simulink model "zadacha_14"  (Simulink 7.1)
settings: Solver=ode45  StartTime=0.0  StopTime=160  RelTol=1e-3
settings Model: Creator=Slavi  LastModifiedBy=Slavi

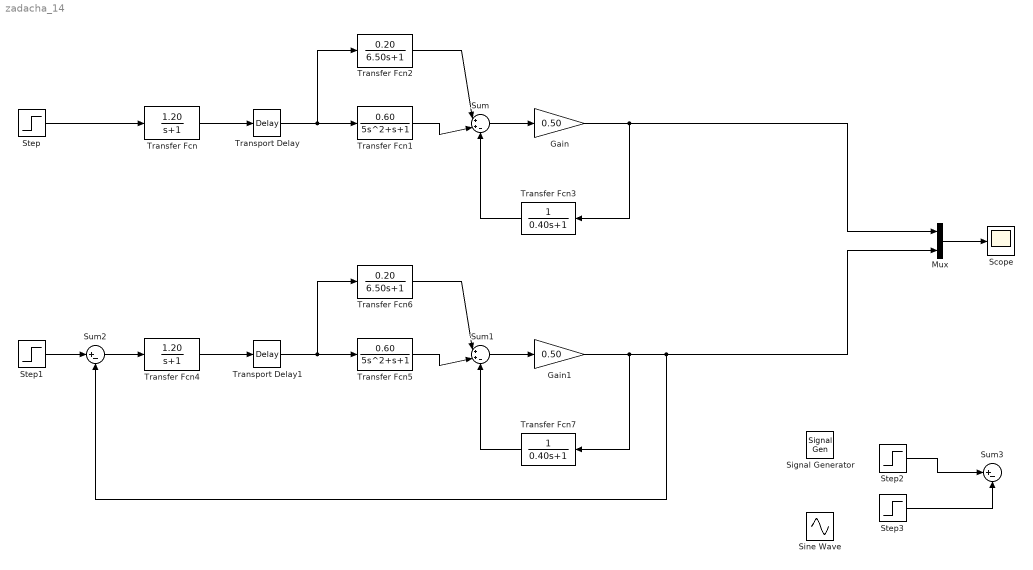
== system zadacha_14 ==
  Gain : Gain  Gain=0.50  ParameterDataType=sfix(16)  ParameterScaling=2^0  OutDataType=sfix(16)  OutScaling=2^0
  Gain1 : Gain  Gain=0.50  ParameterDataType=sfix(16)  ParameterScaling=2^0  OutDataType=sfix(16)  OutScaling=2^0
  Mux : Mux  Inputs=2
  Scope : Scope
  Signal Generator : SignalGenerator
  Sine Wave : Sin
  Step : Step
  Step1 : Step
  Step2 : Step  Time=0
  Step3 : Step
  Sum : Sum  Inputs=|++-  OutDataType=sfix(16)  OutScaling=2^0
  Sum1 : Sum  Inputs=|++-  OutDataType=sfix(16)  OutScaling=2^0
  Sum2 : Sum  Inputs=|+-  OutDataType=sfix(16)  OutScaling=2^0
  Sum3 : Sum  Inputs=|+-  OutDataType=sfix(16)  OutScaling=2^0
  Transfer Fcn : TransferFcn  Numerator=[1.20]  Denominator=[1 1]
  Transfer Fcn1 : TransferFcn  Numerator=[0.60]  Denominator=[5 1 1]
  Transfer Fcn2 : TransferFcn  Numerator=[0.20]  Denominator=[6.50 1]
  Transfer Fcn3 : TransferFcn  Orientation=left  Denominator=[0.40 1]
  Transfer Fcn4 : TransferFcn  Numerator=[1.20]  Denominator=[1 1]
  Transfer Fcn5 : TransferFcn  Numerator=[0.60]  Denominator=[5 1 1]
  Transfer Fcn6 : TransferFcn  Numerator=[0.20]  Denominator=[6.50 1]
  Transfer Fcn7 : TransferFcn  Orientation=left  Denominator=[0.40 1]
  Transport Delay : TransportDelay  DelayTime=2.40
  Transport Delay1 : TransportDelay  DelayTime=2.40
  wires:
  Transfer Fcn/1 -> Transport Delay/1
  Transport Delay/1 -> Transfer Fcn1/1, Transfer Fcn2/1
  Transfer Fcn1/1 -> Sum/2
  Transfer Fcn2/1 -> Sum/1
  Transfer Fcn3/1 -> Sum/3
  Sum/1 -> Gain/1
  Gain/1 -> Transfer Fcn3/1, Mux/1
  Mux/1 -> Scope/1
  Transfer Fcn4/1 -> Transport Delay1/1
  Transport Delay1/1 -> Transfer Fcn5/1, Transfer Fcn6/1
  Transfer Fcn5/1 -> Sum1/2
  Transfer Fcn6/1 -> Sum1/1
  Transfer Fcn7/1 -> Sum1/3
  Sum1/1 -> Gain1/1
  Gain1/1 -> Transfer Fcn7/1, Mux/2, Sum2/2
  Sum2/1 -> Transfer Fcn4/1
  Step2/1 -> Sum3/1
  Step3/1 -> Sum3/2
  Step/1 -> Transfer Fcn/1
  Step1/1 -> Sum2/1
